simulink model "sampleModel1957"  (R2023a)
settings: Solver=VariableStepAuto  StartTime=0.0  StopTime=10.0  RelTol=1e-3
libraries: hdlsllib x4
settings Model: Creator=user1  LastModifiedBy=user1

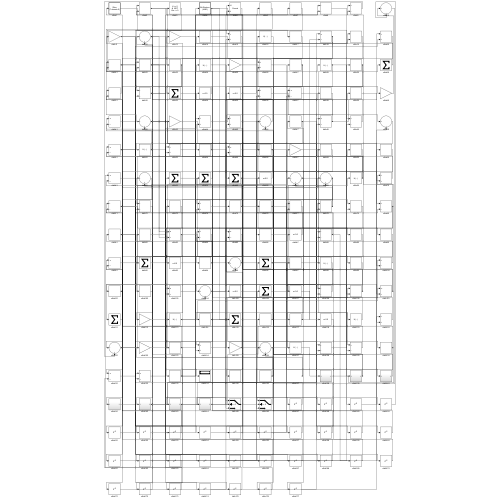
[thumbnail: Simulink's stored preview of the top-level diagram]
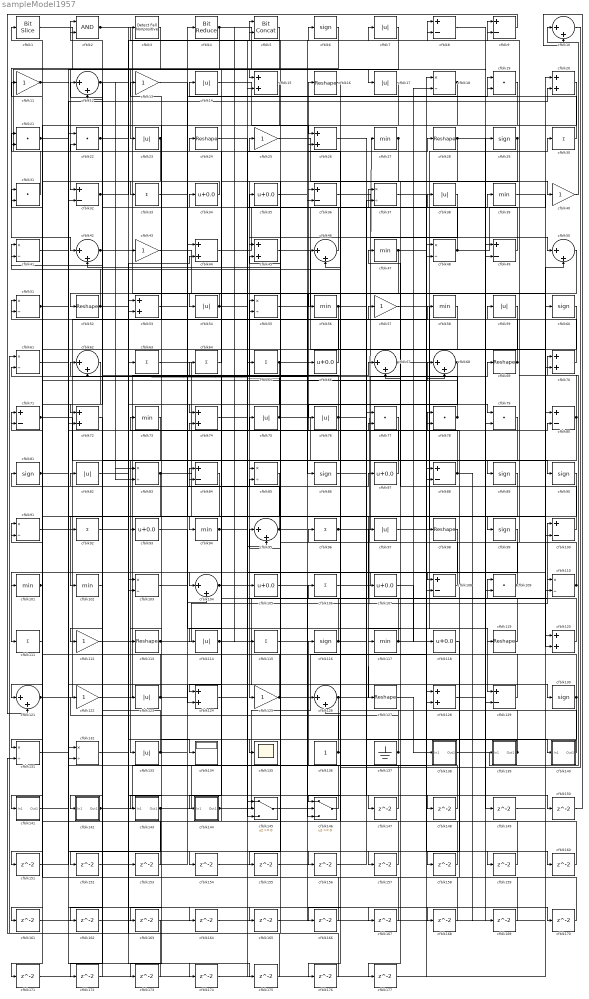
== system sampleModel1957 ==
  cfblk1 : hdlsllib/Logic and Bit Operations/Bit Slice  lidx=7  ridx=0
  cfblk{10,12,42,46,50,62,67..68,95,104,121,126} (12 alike) : Sum  Inputs=|++
  cfblk{8..9,32,36,49,71,80,84,88,100,108,129} (12 alike) : Sum  Inputs=+-
  cfblk{27,39,47,56,58,73,94,101..102,117} (10 alike) : MinMax
  cfblk{18,37,41,48,51,55,61,83,85,91,103,110,131..132} (14 alike) : Product  Inputs=*/  RndMeth=Zero  SaturateOnIntegerOverflow=on
  cfblk{34..35,66,87,93,105,107,118} (8 alike) : Bias  Bias=0.0  SaturateOnIntegerOverflow=off
  cfblk{30,33,63..65,92,96,106,111,115} (10 alike) : Sum  Inputs=+
  cfblk{19,21..22,31,77..79,109} (8 alike) : DotProduct  OutDataTypeStr=Inherit: Inherit via internal rule
  cfblk{11,13,25,40,43,57,112,122,125} (9 alike) : Gain
  cfblk{16,24,28,52,69,98,113,119,127} (9 alike) : Reshape
  cfblk{7,14,17,23,38,54,59,75..76,82,97,114,123,133} (14 alike) : Abs  SaturateOnIntegerOverflow=off
  cfblk{6,29,60,81,86,89..90,99,116,130} (10 alike) : Signum
  cfblk{15,20,26,44..45,53,70,72,74,120,124,128} (12 alike) : Sum
  cfblk134 : Display
  cfblk135 : Scope
  cfblk136 : Constant  SampleTime=-1
  cfblk137 : Ground
  cfblk138 : Subsystem
      settings: LibrarySourceBlock=|
      | hdlsllib/Ports &
      | Subsystems/Subsystem
  cfblk139 : Subsystem
      settings: LibrarySourceBlock=|
      | hdlsllib/Ports &
      | Subsystems/Subsystem
  cfblk140 : Subsystem
      settings: LibrarySourceBlock=|
      | hdlsllib/Ports &
      | Subsystems/Subsystem
  cfblk141 : Subsystem
      settings: LibrarySourceBlock=|
      | hdlsllib/Ports &
      | Subsystems/Subsystem
  cfblk142 : Subsystem
      settings: LibrarySourceBlock=|
      | hdlsllib/Ports &
      | Subsystems/Subsystem
  cfblk143 : Subsystem
      settings: LibrarySourceBlock=|
      | hdlsllib/Ports &
      | Subsystems/Subsystem
  cfblk144 : Subsystem
      settings: LibrarySourceBlock=|
      | hdlsllib/Ports &
      | Subsystems/Subsystem
  cfblk145 : Switch  SaturateOnIntegerOverflow=off  InputSameDT=off
  cfblk146 : Switch  SaturateOnIntegerOverflow=off  InputSameDT=off
  cfblk{147..177} (31 alike) : Delay  SampleTime=1
  cfblk2 : Logic  AllPortsSameDT=off  OutDataTypeStr=boolean
  cfblk3 : hdlsllib/Logic and Bit Operations/Detect Fall Nonpositive  vinit=0  OutDataTypeStr=boolean
  cfblk4 : hdlsllib/Logic and Bit Operations/Bit Reduce  mode=AND
  cfblk5 : hdlsllib/Logic and Bit Operations/Bit Concat  numInputs=2
  wires:
  cfblk77/1 -> cfblk133/1
  cfblk142/1(Out1) -> cfblk116/1, cfblk88/1
  cfblk98/1 -> cfblk111/1
  cfblk54/1 -> cfblk52/1, cfblk110/2
  cfblk126/1 -> cfblk27/1, cfblk146/3
  cfblk29/1 -> cfblk125/1, cfblk79/2
  cfblk107/1 -> cfblk118/1
  cfblk99/1 -> cfblk101/1
  cfblk42/1 -> cfblk54/1, cfblk70/2, cfblk43/1
  cfblk127/1 -> cfblk138/1(In1)
  cfblk130/1 -> cfblk62/1, cfblk173/1
  cfblk122/1 -> cfblk67/1
  cfblk57/1 -> cfblk129/1
  cfblk97/1 -> cfblk30/1
  cfblk121/1 -> cfblk55/1, cfblk159/1
  cfblk44/1 -> cfblk38/1
  cfblk21/1 -> cfblk167/1, cfblk168/1
  cfblk73/1 -> cfblk93/1
  cfblk55/1 -> cfblk39/1
  cfblk129/1 -> cfblk96/1
  cfblk112/1 -> cfblk123/1
  cfblk69/1 -> cfblk35/1, cfblk47/1
  cfblk87/1 -> cfblk16/1
  cfblk27/1 -> cfblk104/1, cfblk135/1
  cfblk104/1 -> cfblk105/1, cfblk7/1
  cfblk76/1 -> cfblk41/1, cfblk90/1, cfblk155/1
  cfblk91/1 -> cfblk66/1
  cfblk120/1 -> cfblk36/1
  cfblk31/1 -> cfblk17/1
  cfblk84/1 -> cfblk102/1
  cfblk51/1 -> cfblk94/1, cfblk174/1
  cfblk139/1(Out1) -> cfblk73/1, cfblk61/2
  cfblk65/1 -> cfblk79/1, cfblk163/1
  cfblk67/1 -> cfblk68/2, cfblk177/1
  cfblk47/1 -> cfblk85/1, cfblk160/1
  cfblk96/1 -> cfblk69/1, cfblk140/1(In1)
  cfblk63/1 -> cfblk95/2
  cfblk50/1 -> cfblk53/2
  cfblk124/1 -> cfblk58/1
  cfblk133/1 -> cfblk82/1, cfblk8/1, cfblk5/1
  cfblk128/1 -> cfblk29/1
  cfblk93/1 -> cfblk119/1
  cfblk62/1 -> cfblk121/1
  cfblk6/1 -> cfblk42/1
  cfblk109/1 -> cfblk42/2, cfblk21/2
  cfblk43/1 -> cfblk98/1
  cfblk2/1 -> cfblk86/1, cfblk175/1
  cfblk3/1 -> cfblk32/1
  cfblk132/1 -> cfblk44/2
  cfblk114/1 -> cfblk129/2, cfblk48/1
  cfblk14/1 -> cfblk26/1
  cfblk100/1 -> cfblk57/1
  cfblk78/1 -> cfblk55/2, cfblk51/1
  cfblk115/1 -> cfblk19/1
  cfblk116/1 -> cfblk81/1, cfblk109/1
  cfblk32/1 -> cfblk8/2, cfblk148/1
  cfblk7/1 -> cfblk23/1
  cfblk30/1 -> cfblk14/1
  cfblk48/1 -> cfblk20/1, cfblk2/2
  cfblk15/1 -> cfblk132/2
  cfblk101/1 -> cfblk71/1, cfblk151/1
  cfblk11/1 -> cfblk156/1, cfblk157/1
  cfblk138/1(Out1) -> cfblk70/1
  cfblk125/1 -> cfblk91/1, cfblk68/1
  cfblk144/1(Out1) -> cfblk18/1, cfblk110/1
  cfblk60/1 -> cfblk67/2
  cfblk10/1 -> cfblk126/2
  cfblk110/1 -> cfblk9/1, cfblk3/1
  cfblk90/1 -> cfblk127/1
  cfblk113/1 -> cfblk100/1, cfblk6/1
  cfblk20/1 -> cfblk124/1
  cfblk36/1 -> cfblk50/1
  cfblk23/1 -> cfblk32/2, cfblk131/1
  cfblk92/1 -> cfblk63/1
  cfblk35/1 -> cfblk9/2
  cfblk9/1 -> cfblk121/2
  cfblk72/1 -> cfblk142/1(In1)
  cfblk89/1 -> cfblk141/1(In1)
  cfblk37/1 -> cfblk100/2
  cfblk106/1 -> cfblk108/1
  cfblk103/1 -> cfblk87/1
  cfblk66/1 -> cfblk13/1
  cfblk83/1 -> cfblk108/2, cfblk112/1
  cfblk75/1 -> cfblk139/1(In1), cfblk62/2
  cfblk46/1 -> cfblk12/1
  cfblk22/1 -> cfblk134/1, cfblk128/2, cfblk83/1
  cfblk40/1 -> cfblk10/1
  cfblk1/1 -> cfblk15/1
  cfblk49/1 -> cfblk25/1
  cfblk143/1(Out1) -> cfblk145/2, cfblk88/2, cfblk172/1
  cfblk131/1 -> cfblk75/1
  cfblk45/1 -> cfblk120/2
  cfblk52/1 -> cfblk31/2, cfblk165/1
  cfblk13/1 -> cfblk99/1
  cfblk5/1 -> cfblk74/1
  cfblk25/1 -> cfblk40/1
  cfblk38/1 -> cfblk45/1
  cfblk102/1 -> cfblk22/2
  cfblk137/1 -> cfblk122/1, cfblk51/2
  cfblk16/1 -> cfblk56/1
  cfblk74/1 -> cfblk37/1
  cfblk86/1 -> cfblk78/1
  cfblk18/1 -> cfblk146/1, cfblk113/1
  cfblk28/1 -> cfblk117/1, cfblk130/1
  cfblk53/1 -> cfblk4/1
  cfblk68/1 -> cfblk103/2, cfblk144/1(In1)
  cfblk123/1 -> cfblk19/2, cfblk143/1(In1), cfblk21/1
  cfblk70/1 -> cfblk11/1
  cfblk140/1(Out1) -> cfblk41/2
  cfblk64/1 -> cfblk24/1
  cfblk111/1 -> cfblk31/1
  cfblk108/1 -> cfblk34/1
  cfblk95/1 -> cfblk84/1, cfblk80/2
  cfblk80/1 -> cfblk59/1, cfblk145/3, cfblk107/1
  cfblk71/1 -> cfblk145/1, cfblk77/2
  cfblk136/1 -> cfblk106/1, cfblk2/1
  cfblk24/1 -> cfblk65/1
  cfblk59/1 -> cfblk76/1
  cfblk56/1 -> cfblk114/1, cfblk109/2, cfblk176/1
  cfblk61/1 -> cfblk92/1
  cfblk117/1 -> cfblk46/2, cfblk18/2
  cfblk94/1 -> cfblk64/1, cfblk28/1
  cfblk119/1 -> cfblk97/1
  cfblk88/1 -> cfblk26/2, cfblk169/1
  cfblk4/1 -> cfblk49/1, cfblk72/2, cfblk115/1
  cfblk12/1 -> cfblk72/1, cfblk83/2, cfblk164/1
  cfblk81/1 -> cfblk20/2, cfblk124/2
  cfblk146/1 -> cfblk85/2
  cfblk34/1 -> cfblk33/1
  cfblk33/1 -> cfblk89/1
  cfblk145/1 -> cfblk146/2
  cfblk39/1 -> cfblk80/1
  cfblk105/1 -> cfblk147/1
  cfblk147/1 -> cfblk44/1
  cfblk148/1 -> cfblk132/1
  cfblk8/1 -> cfblk149/1
  cfblk149/1 -> cfblk50/2
  cfblk26/1 -> cfblk150/1
  cfblk150/1 -> cfblk10/2
  cfblk151/1 -> cfblk22/1
  cfblk85/1 -> cfblk152/1
  cfblk152/1 -> cfblk104/2
  cfblk82/1 -> cfblk153/1
  cfblk153/1 -> cfblk91/2
  cfblk41/1 -> cfblk154/1
  cfblk154/1 -> cfblk37/2
  cfblk155/1 -> cfblk5/2
  cfblk156/1 -> cfblk77/1
  cfblk157/1 -> cfblk71/2
  cfblk118/1 -> cfblk158/1
  cfblk158/1 -> cfblk126/1
  cfblk159/1 -> cfblk84/2
  cfblk160/1 -> cfblk74/2
  cfblk58/1 -> cfblk161/1
  cfblk161/1 -> cfblk120/1
  cfblk79/1 -> cfblk162/1
  cfblk162/1 -> cfblk36/2
  cfblk163/1 -> cfblk131/2
  cfblk164/1 -> cfblk49/2
  cfblk165/1 -> cfblk46/1
  cfblk17/1 -> cfblk166/1
  cfblk166/1 -> cfblk103/1
  cfblk167/1 -> cfblk95/1
  cfblk168/1 -> cfblk1/1
  cfblk169/1 -> cfblk78/2
  cfblk141/1(Out1) -> cfblk170/1
  cfblk170/1 -> cfblk128/1
  cfblk19/1 -> cfblk171/1
  cfblk171/1 -> cfblk15/2
  cfblk172/1 -> cfblk12/2
  cfblk173/1 -> cfblk53/1
  cfblk174/1 -> cfblk48/2
  cfblk175/1 -> cfblk61/1
  cfblk176/1 -> cfblk45/2
  cfblk177/1 -> cfblk60/1

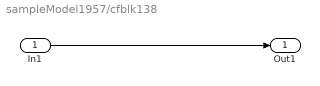
== system sampleModel1957/cfblk138 ==
  In1 : Inport
  Out1 : Outport
  wires:
  In1/1 -> Out1/1

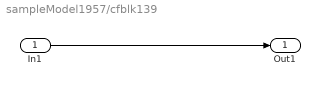
== system sampleModel1957/cfblk139 ==
  In1 : Inport
  Out1 : Outport
  wires:
  In1/1 -> Out1/1

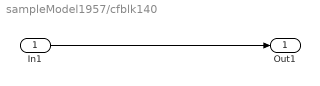
== system sampleModel1957/cfblk140 ==
  In1 : Inport
  Out1 : Outport
  wires:
  In1/1 -> Out1/1

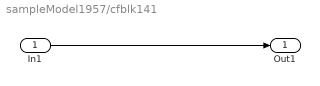
== system sampleModel1957/cfblk141 ==
  In1 : Inport
  Out1 : Outport
  wires:
  In1/1 -> Out1/1

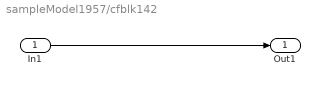
== system sampleModel1957/cfblk142 ==
  In1 : Inport
  Out1 : Outport
  wires:
  In1/1 -> Out1/1

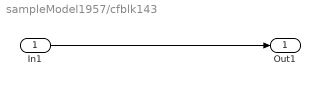
== system sampleModel1957/cfblk143 ==
  In1 : Inport
  Out1 : Outport
  wires:
  In1/1 -> Out1/1

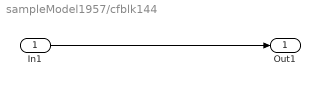
== system sampleModel1957/cfblk144 ==
  In1 : Inport
  Out1 : Outport
  wires:
  In1/1 -> Out1/1
